simulink model "lookup_nD_TestGen42"  (R2017b)
settings: Solver=FixedStepDiscrete  StartTime=0.0  StopTime=10.0  RelTol=1e-3
model workspace (MAT data in the model file):
  LUTObjLKnD42 = Simulink.LookupTable
  LUTObjLKnD42.Table = Simulink.lookuptable.Table
  LUTObjLKnD42.Table.Value = [4 16 10 4 16 10 4 16 10 4 16 10 ... (2160 elements, 2x5x3x2x3x4x3)]
  LUTObjLKnD42.Table.Dimensions = [2 5 3 2 3 4 3]
  LUTObjLKnD42.Table.DataType = 'auto'
  LUTObjLKnD42.Table.FieldName = 'Table'
  LUTObjLKnD42.BreakpointsSpecification = 'Even spacing'
  LUTObjLKnD42.Breakpoints(1) = Simulink.lookuptable.Evenspacing
  LUTObjLKnD42.Breakpoints(1).FirstPoint = 63.9361709448
  LUTObjLKnD42.Breakpoints(1).Spacing = 1.5
  LUTObjLKnD42.Breakpoints(1).FirstPointName = 'BPFirstPoint1'
  LUTObjLKnD42.Breakpoints(1).SpacingName = 'BPSpacing1'
  LUTObjLKnD42.Breakpoints(1).TunableSizeName = 'N1'
  LUTObjLKnD42.Breakpoints(1).DataType = 'auto'
  LUTObjLKnD42.Breakpoints(1).FieldName = 'BP1'
  LUTObjLKnD42.Breakpoints(2) = Simulink.lookuptable.Evenspacing
  LUTObjLKnD42.Breakpoints(2).FirstPoint = 3.99182837967
  LUTObjLKnD42.Breakpoints(2).Spacing = 1.5
  LUTObjLKnD42.Breakpoints(2).FirstPointName = 'BPFirstPoint2'
  LUTObjLKnD42.Breakpoints(2).SpacingName = 'BPSpacing2'
  LUTObjLKnD42.Breakpoints(2).TunableSizeName = 'N2'
  LUTObjLKnD42.Breakpoints(2).DataType = 'auto'
  LUTObjLKnD42.Breakpoints(2).FieldName = 'BP2'
  LUTObjLKnD42.Breakpoints(3) = Simulink.lookuptable.Evenspacing
  LUTObjLKnD42.Breakpoints(3).FirstPoint = 96.9448546336
  LUTObjLKnD42.Breakpoints(3).Spacing = 1.5
  LUTObjLKnD42.Breakpoints(3).FirstPointName = 'BPFirstPoint3'
  LUTObjLKnD42.Breakpoints(3).SpacingName = 'BPSpacing3'
  LUTObjLKnD42.Breakpoints(3).TunableSizeName = 'N3'
  LUTObjLKnD42.Breakpoints(3).DataType = 'auto'
  LUTObjLKnD42.Breakpoints(3).FieldName = 'BP3'
  LUTObjLKnD42.Breakpoints(4) = Simulink.lookuptable.Evenspacing
  LUTObjLKnD42.Breakpoints(4).FirstPoint = 99.9288288542
  LUTObjLKnD42.Breakpoints(4).Spacing = 1.5
  LUTObjLKnD42.Breakpoints(4).FirstPointName = 'BPFirstPoint4'
  LUTObjLKnD42.Breakpoints(4).SpacingName = 'BPSpacing4'
  LUTObjLKnD42.Breakpoints(4).TunableSizeName = 'N4'
  LUTObjLKnD42.Breakpoints(4).DataType = 'auto'
  LUTObjLKnD42.Breakpoints(4).FieldName = 'BP4'
  LUTObjLKnD42.Breakpoints(5) = Simulink.lookuptable.Evenspacing
  LUTObjLKnD42.Breakpoints(5).FirstPoint = 104.638803787
  LUTObjLKnD42.Breakpoints(5).Spacing = 1.5
  LUTObjLKnD42.Breakpoints(5).FirstPointName = 'BPFirstPoint5'
  LUTObjLKnD42.Breakpoints(5).SpacingName = 'BPSpacing5'
  LUTObjLKnD42.Breakpoints(5).TunableSizeName = 'N5'
  LUTObjLKnD42.Breakpoints(5).DataType = 'auto'
  LUTObjLKnD42.Breakpoints(5).FieldName = 'BP5'
  LUTObjLKnD42.Breakpoints(6) = Simulink.lookuptable.Evenspacing
  LUTObjLKnD42.Breakpoints(6).FirstPoint = 48.6214501523
  LUTObjLKnD42.Breakpoints(6).Spacing = 1.5
  LUTObjLKnD42.Breakpoints(6).FirstPointName = 'BPFirstPoint6'
  LUTObjLKnD42.Breakpoints(6).SpacingName = 'BPSpacing6'
  LUTObjLKnD42.Breakpoints(6).TunableSizeName = 'N6'
  LUTObjLKnD42.Breakpoints(6).DataType = 'auto'
  LUTObjLKnD42.Breakpoints(6).FieldName = 'BP6'
  LUTObjLKnD42.Breakpoints(7) = Simulink.lookuptable.Evenspacing
  LUTObjLKnD42.Breakpoints(7).FirstPoint = 44.9081042164
  LUTObjLKnD42.Breakpoints(7).Spacing = 1.5
  LUTObjLKnD42.Breakpoints(7).FirstPointName = 'BPFirstPoint7'
  LUTObjLKnD42.Breakpoints(7).SpacingName = 'BPSpacing7'
  LUTObjLKnD42.Breakpoints(7).TunableSizeName = 'N7'
  LUTObjLKnD42.Breakpoints(7).DataType = 'auto'
  LUTObjLKnD42.Breakpoints(7).FieldName = 'BP7'
  LUTObjLKnD42.SupportTunableSize = 0
  LUTObjLKnD42.StructTypeInfo = Simulink.lookuptable.StructTypeInfo
  LUTObjLKnD42.StructTypeInfo.Name = 'LUT'
  LUTObjLKnD42.StructTypeInfo.DataScope = 'Auto'
settings Model: Creator=ktrinh  LastModifiedBy=ktrinh
settings DebuggingCC: ParameterOverflowMsg=none

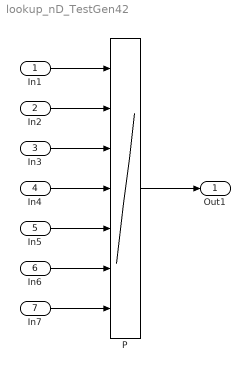
== system lookup_nD_TestGen42 ==
  In1 : Inport  OutMin=0  OutMax=127  PortDimensions=1
  In2 : Inport  Port=2  OutMin=0  OutMax=127
  In3 : Inport  Port=3  OutMin=0  OutMax=127
  In4 : Inport  Port=4  OutMin=0  OutMax=127
  In5 : Inport  Port=5  OutMin=0  OutMax=127
  In6 : Inport  Port=6  OutMin=0  OutMax=127
  In7 : Inport  Port=7  OutMin=0  OutMax=127
  P : Lookup_n-D  NumberOfTableDimensions=7  DataSpecification=Lookup table object  LookupTableObject=LUTObjLKnD42  BreakpointsSpecification=Even spacing  BreakpointsForDimension3=[5, 7]  Table=reshape(repmat([4 5 6;16 19 20;10 18 23],1,2),[3,3,2])  InternalRulePriority=Speed  RndMeth=Simplest  InputSameDT=on
  Out1 : Outport
  wires:
  In1/1 -> P/1
  In2/1 -> P/2
  In3/1 -> P/3
  In4/1 -> P/4
  In5/1 -> P/5
  In6/1 -> P/6
  In7/1 -> P/7
  P/1 -> Out1/1
